simulink subsystem "rss_MotoSTMSens"  (R2023a)
settings: Solver=VariableStepAuto  StartTime=0.0  StopTime=10.0  RelTol=1e-3
undefined symbols (not defined in the file): Cdbl_nElecAgSpdMaxVal
settings Model: Creator=xiaoqiang.yuan  LastModifiedBy=xiaoqiang.yuan

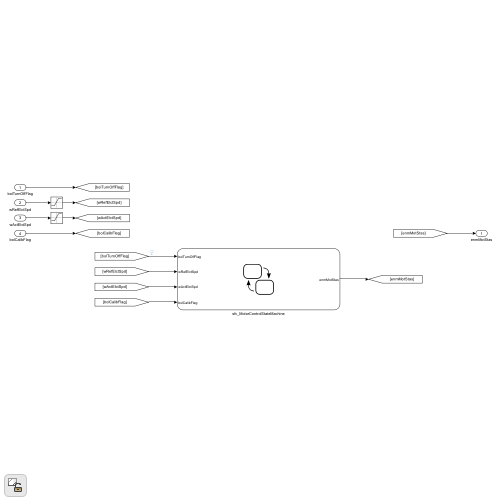
[thumbnail: Simulink's stored preview of the top-level diagram]
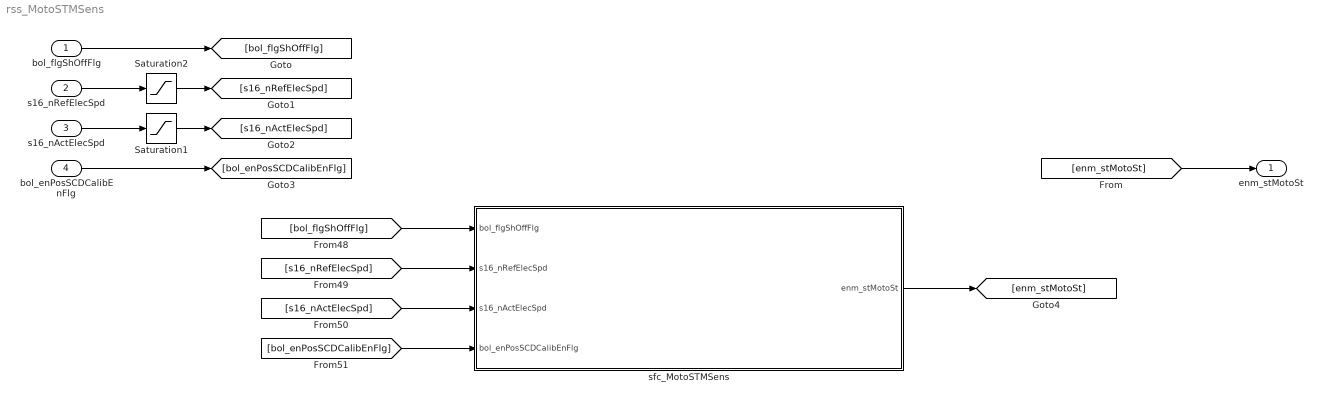
== system rss_MotoSTMSens ==
  bol_flgShOffFlg : Inport  OutDataTypeStr=boolean
  s16_nRefElecSpd : Inport  Port=2  OutDataTypeStr=dt_Standardize_s16p15b0
  s16_nActElecSpd : Inport  Port=3  OutDataTypeStr=dt_Standardize_s16p15b0
  bol_enPosSCDCalibEnFlg : Inport  Port=4  OutDataTypeStr=boolean
  Saturation1 : Saturate  UpperLimit=Cdbl_nElecAgSpdMaxVal  LowerLimit=-Cdbl_nElecAgSpdMaxVal
  Saturation2 : Saturate  UpperLimit=Cdbl_nElecAgSpdMaxVal  LowerLimit=-Cdbl_nElecAgSpdMaxVal
  sfc_MotoSTMSens : Stateflow chart  TreatAsAtomicUnit=on
  enm_stMotoSt : Outport  OutDataTypeStr=Enum: ENM_MOTO_STATUS
  wires:
  [bol_flgShOffFlg] -> sfc_MotoSTMSens/1(bol_flgShOffFlg)
  [s16_nRefElecSpd] -> sfc_MotoSTMSens/2(s16_nRefElecSpd)
  [s16_nActElecSpd] -> sfc_MotoSTMSens/3(s16_nActElecSpd)
  [bol_enPosSCDCalibEnFlg] -> sfc_MotoSTMSens/4(bol_enPosSCDCalibEnFlg)
  bol_flgShOffFlg/1 -> [bol_flgShOffFlg]
  s16_nRefElecSpd/1 -> Saturation2/1
  s16_nActElecSpd/1 -> Saturation1/1
  bol_enPosSCDCalibEnFlg/1 -> [bol_enPosSCDCalibEnFlg]
  Saturation2/1 -> [s16_nRefElecSpd]
  Saturation1/1 -> [s16_nActElecSpd]
  sfc_MotoSTMSens/1(enm_stMotoSt) -> [enm_stMotoSt]
  [enm_stMotoSt] -> enm_stMotoSt/1

== stateflow chart rss_MotoSTMSens/sfc_MotoSTMSens ==
  state OFF
    en:
    enm_stMotoSt = ENM_MOTO_STATUS.OFF;
  state CLOSED_LOOP
    en:
    enm_stMotoSt = ENM_MOTO_STATUS.CLOSED_LOOP;
  (default) -> OFF
  (junction 14) -> OFF
  CLOSED_LOOP -> (junction 14) : [(s16_nRefElecSpd == 0 && ...
      | abs(s16_nActElecSpd) < abs(Gs16_nShOffActElecSpd_C) &&...
      | not(bol_enPosSCDCalibEnFlg)) || ...
      | bol_flgShOffFlg]
  OFF -> (junction 6) : [(abs(s16_nRefElecSpd) > 0 || ...
      | bol_enPosSCDCalibEnFlg ) && ...
      | not(bol_flgShOffFlg)]
  (junction 6) -> CLOSED_LOOP
  data: bol_flgShOffFlg input boolean; s16_nRefElecSpd input dt_Standardize_s16p15b0; s16_nActElecSpd input dt_Standardize_s16p15b0; bol_enPosSCDCalibEnFlg input boolean; enm_stMotoSt output Enum: ENM_MOTO_STATUS; Gs16_nShOffActElecSpd_C parameter
